simulink model "PI_Controller"  (R2019a)
settings: Solver=VariableStepAuto  StartTime=0.0  StopTime=50  RelTol=1e-3
undefined symbols (not defined in the file): G1, G2, Ki, Kp
settings Model: Creator=Gabe Casciano  LastModifiedBy=Gabe Casciano

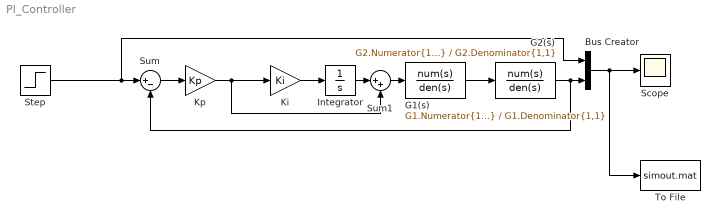
== system PI_Controller ==
  Bus Creator : BusCreator  Inputs=2
  G1(s) : TransferFcn  Numerator=G1.Numerator{1,1}  Denominator=G1.Denominator{1,1}
  G2(s) : TransferFcn  Numerator=G2.Numerator{1,1}  Denominator=G2.Denominator{1,1}
  Integrator : Integrator
  Ki : Gain  Gain=Ki
  Kp : Gain  Gain=Kp
  Scope : Scope
  Step : Step  SampleTime=0
  Sum : Sum  Inputs=|+-
  Sum1 : Sum  Inputs=|++
  To File : ToFile  Filename=simout.mat  SaveFormat=Timeseries
  wires:
  Step/1 -> Bus Creator/1, Sum/1
  G2(s)/1 -> Sum/2, Bus Creator/2
  Sum/1 -> Kp/1
  G1(s)/1 -> G2(s)/1
  Bus Creator/1 -> To File/1, Scope/1
  Sum1/1 -> G1(s)/1
  Kp/1 -> Sum1/2, Ki/1
  Ki/1 -> Integrator/1
  Integrator/1 -> Sum1/1
